simulink model "final"  (R2020a)
settings: Solver=FixedStepAuto  StartTime=0.0  StopTime=10.0  FixedStep=0.0001  RelTol=1e-3
values from neighbouring files (symbols this model uses):
  A = [0 0  1 0 ... (first row only)    [Robust_control_Lyapunov.m]
  alpha = max(abs(dm))    [Robust_control_Lyapunov.m]
  b = [1 ... (first row only)    [Robust_control_Lyapunov.m]
  K = place(A,b,pole)    [Robust_control_Lyapunov.m]
  P = lyap(Ac',Q)    [Robust_control_Lyapunov.m]
settings Model: Creator=楊士賢  LastModifiedBy=楊士賢

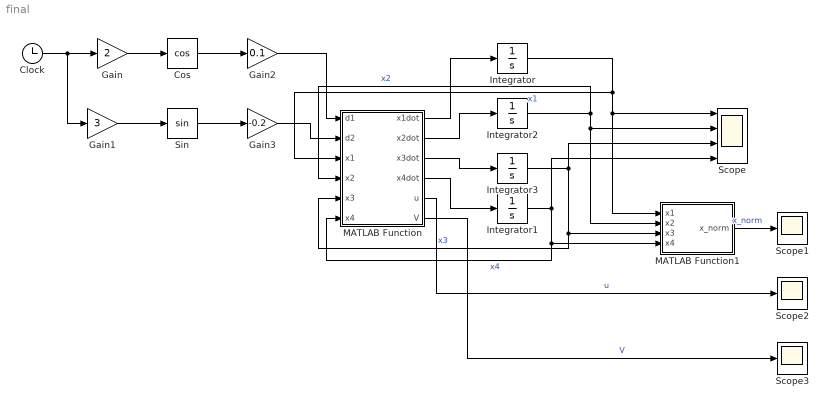
== system final ==
  Clock : Clock
  Cos : Trigonometry  Operator=cos
  Gain : Gain  Gain=2
  Gain1 : Gain  Gain=3
  Gain2 : Gain  Gain=0.1
  Gain3 : Gain  Gain=-0.2
  Integrator : Integrator  InitialCondition=5
  Integrator1 : Integrator
  Integrator2 : Integrator
  Integrator3 : Integrator  InitialCondition=-6
  MATLAB Function : MATLAB Function  TreatAsAtomicUnit=on
  MATLAB Function1 : MATLAB Function  TreatAsAtomicUnit=on
  Scope : Scope  NumInputPorts=4
  Scope1 : Scope
  Scope2 : Scope
  Scope3 : Scope
  Sin : Trigonometry
  wires:
  Integrator/1 -> MATLAB Function1/1(x1), Scope/1, MATLAB Function/3(x1)  "x1"
  MATLAB Function/1(x1dot) -> Integrator/1
  MATLAB Function/4(x4dot) -> Integrator1/1
  MATLAB Function/2(x2dot) -> Integrator2/1
  MATLAB Function/3(x3dot) -> Integrator3/1
  Integrator2/1 -> MATLAB Function1/2(x2), Scope/2, MATLAB Function/4(x2)  "x2"
  Integrator3/1 -> Scope/3, MATLAB Function1/3(x3), MATLAB Function/5(x3)  "x3"
  Integrator1/1 -> Scope/4, MATLAB Function/6(x4), MATLAB Function1/4(x4)  "x4"
  Clock/1 -> Gain1/1, Gain/1
  Gain/1 -> Cos/1
  Gain1/1 -> Sin/1
  Sin/1 -> Gain3/1
  Cos/1 -> Gain2/1
  Gain2/1 -> MATLAB Function/1(d1)
  Gain3/1 -> MATLAB Function/2(d2)
  MATLAB Function1/1(x_norm) -> Scope1/1  "x_norm"
  MATLAB Function/5(u) -> Scope2/1  "u"
  MATLAB Function/6(V) -> Scope3/1  "V"

== matlab function final/MATLAB Function1 ==
  data: x1 input; x_norm output; x2 input; x3 input; x4 input
function x_norm = fcn(x1,x2,x3,x4)

X = [x1 x2 x3 x4]';
x_norm = norm(X);

== matlab function final/MATLAB Function ==
  data: d1 input; d2 input; x1 input; x1dot output; x2dot output; x3dot output; x4dot output; x2 input; x3 input; x4 input; E parameter; b parameter; A parameter; alpha parameter; P parameter; K parameter; u output; V output
function [x1dot,x2dot,x3dot,x4dot,u,V] = fcn(d1, d2, x1,x2,x3,x4, E, b, A,alpha, P,K)
d = [d1;d2];
X = [x1 x2 x3 x4]';
u = -K*X-alpha*b'*P*X/norm(b'*P*X);
x_dot = A*X+b*u+E*d;

V = 1/2*X'*P*X;
x1dot = x_dot(1);
x2dot = x_dot(2);
x3dot = x_dot(3);
x4dot= x_dot(4);
